simulink model "FMS_TECS"  (R2022b)
settings: Solver=FixedStepDiscrete  StartTime=0.0  StopTime=10.0  FixedStep=CONTROL_CONST.dt  RelTol=1e-3
values from neighbouring files (symbols this model uses):
  CONTROL_PARAM = Simulink.Parameter(CONTROL_PARAM_VALUE)    [control_model_init.m]
undefined symbols (not defined in the file or in its folder): CONTROL_CONST, CONTROL_PARAM_VALUE, DiscIntNeverNeededParam
libraries: FC_Lib x5, simulink x1, aerolibasang x1
settings Model: Creator=19114  LastModifiedBy=19114
settings OptimizationCC: DefaultParameterBehavior=Inlined  DefaultUnderspecifiedDataType=single  EnhancedBackFolding=on  PassReuseOutputArgsAs=Individual arguments  ZeroExternalMemoryAtStartup=off  ZeroInternalMemoryAtStartup=off  OptimizeBlockOrder=speed  DifferentSizesBufferReuse=on  OptimizationCustomize=off  EfficientTunableParamExpr=on
settings DebuggingCC: ParameterTunabilityLossMsg=error
settings HardwareCC: ProdBitPerLong=64  ProdLongLongMode=on  ProdHWDeviceType=Intel->x86-64 (Linux 64)
settings SFSimCC: MATLABDynamicMemAlloc=off
settings RTWCC: Description=Embedded Coder  SystemTargetFile=ert.tlc  GenCodeOnly=on  TemplateMakefile=ert_default_tmf  TargetLang=C++
settings CodeAppCC: ForceParamTrailComments=on  IgnoreCustomStorageClasses=off  OperatorAnnotations=on  SimulinkDataObjDesc=on  SFDataObjDesc=on  InsertBlockDesc=on
settings ERTTargetCC: TargetLangStandard=C++11 (ISO)  GenerateSampleERTMain=on  CodeInterfacePackaging=C++ class  InlinedParameterPlacement=NonHierarchical  RootIOFormat=Structure reference  ERTCustomFileTemplate=example_file_process.tlc

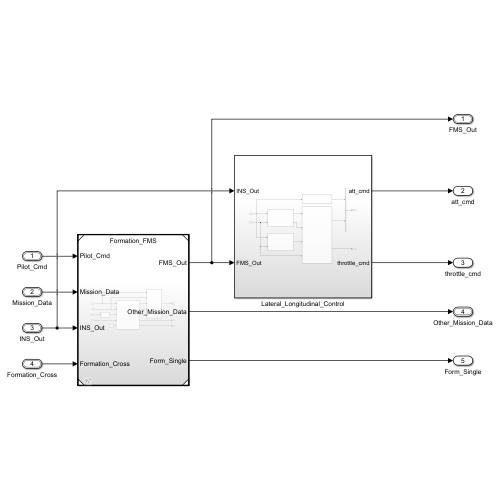
[thumbnail: Simulink's stored preview of the top-level diagram]
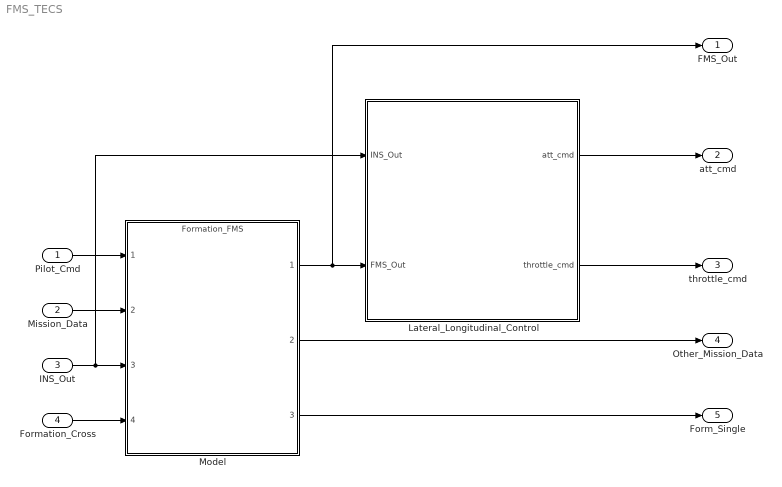
== system FMS_TECS ==
  Pilot_Cmd : Inport  OutDataTypeStr=Bus: Pilot_Cmd_Bus
  Mission_Data : Inport  Port=2  OutDataTypeStr=Bus: Mission_Data_Bus
  INS_Out : Inport  Port=3  OutDataTypeStr=Bus: INS_Out_Bus
  Formation_Cross : Inport  Port=4  OutDataTypeStr=Bus: Formation_Cross_Bus
  Lateral_Longitudinal_Control : Subsystem
  Model : ModelReference  ModelNameDialog=Formation_FMS.slx  SimulationMode=Normal  ModelReferenceVersion=1.179
  FMS_Out : Outport  OutDataTypeStr=Bus: FMS_Out_Bus  VectorParamsAs1DForOutWhenUnconnected=off
  att_cmd : Outport  Port=2
  throttle_cmd : Outport  Port=3
  Other_Mission_Data : Outport  Port=4  OutDataTypeStr=Bus: Other_Mission_Data_Bus  VectorParamsAs1DForOutWhenUnconnected=off
  Form_Single : Outport  Port=5
  wires:
  Lateral_Longitudinal_Control/1(att_cmd) -> att_cmd/1
  Lateral_Longitudinal_Control/2(throttle_cmd) -> throttle_cmd/1
  Pilot_Cmd/1 -> Model/1
  Mission_Data/1 -> Model/2
  INS_Out/1 -> Lateral_Longitudinal_Control/1(INS_Out), Model/3
  Formation_Cross/1 -> Model/4
  Model/1 -> FMS_Out/1, Lateral_Longitudinal_Control/2(FMS_Out)
  Model/2 -> Other_Mission_Data/1
  Model/3 -> Form_Single/1

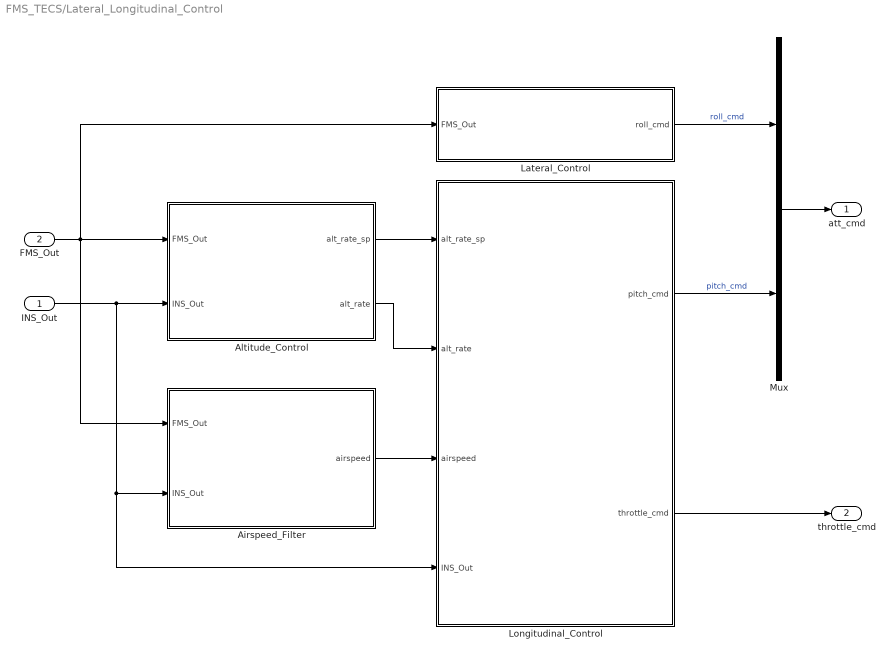
== system FMS_TECS/Lateral_Longitudinal_Control ==
  INS_Out : Inport
  FMS_Out : Inport  Port=2
  Airspeed_Filter : Subsystem
  Altitude_Control : Subsystem
  Lateral_Control : Subsystem
  Longitudinal_Control : Subsystem
  Mux : Mux  Inputs=2
  att_cmd : Outport  VectorParamsAs1DForOutWhenUnconnected=off
  throttle_cmd : Outport  Port=2  VectorParamsAs1DForOutWhenUnconnected=off
  wires:
  FMS_Out/1 -> Lateral_Control/1(FMS_Out), Airspeed_Filter/1(FMS_Out), Altitude_Control/1(FMS_Out)
  Altitude_Control/1(alt_rate_sp) -> Longitudinal_Control/1(alt_rate_sp)
  INS_Out/1 -> Longitudinal_Control/4(INS_Out), Airspeed_Filter/2(INS_Out), Altitude_Control/2(INS_Out)
  Longitudinal_Control/1(pitch_cmd) -> Mux/2  "pitch_cmd"
  Altitude_Control/2(alt_rate) -> Longitudinal_Control/2(alt_rate)
  Longitudinal_Control/2(throttle_cmd) -> throttle_cmd/1
  Airspeed_Filter/1(airspeed) -> Longitudinal_Control/3(airspeed)
  Lateral_Control/1(roll_cmd) -> Mux/1  "roll_cmd"
  Mux/1 -> att_cmd/1

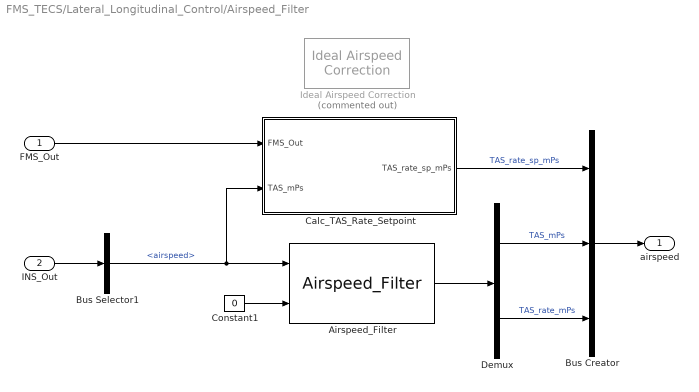
== system FMS_TECS/Lateral_Longitudinal_Control/Airspeed_Filter ==
  FMS_Out : Inport
  INS_Out : Inport  Port=2
  Airspeed_Filter : FC_Lib/Control/Airspeed_Filter
      settings: SourceProductName=Flight Control Toolbox
  Bus Creator : BusCreator  Inputs=3
  Bus Selector1 : BusSelector  OutputSignals=airspeed
  Calc_TAS_Rate_Setpoint : Subsystem
  Constant1 : Constant  Value=0  OutDataTypeStr=single
  Demux : Demux  Outputs=2
  Ideal Airspeed Correction : aerolibasang/Ideal Airspeed Correction  Commented=on  units=Metric (MKS)  vel_in=CAS  vel_out_tas=CAS  vel_out_eas=TAS  vel_out_cas=TAS  method=Table Lookup  SubOnly=on  action=None
  airspeed : Outport
  wires:
  INS_Out/1 -> Bus Selector1/1
  Bus Creator/1 -> airspeed/1
  Bus Selector1/1 -> Calc_TAS_Rate_Setpoint/2(TAS_mPs), Airspeed_Filter/1  "<airspeed>"
  FMS_Out/1 -> Calc_TAS_Rate_Setpoint/1(FMS_Out)
  Calc_TAS_Rate_Setpoint/1(TAS_rate_sp_mPs) -> Bus Creator/1  "TAS_rate_sp_mPs"
  Demux/1 -> Bus Creator/2  "TAS_mPs"
  Demux/2 -> Bus Creator/3  "TAS_rate_mPs"
  Airspeed_Filter/1 -> Demux/1
  Constant1/1 -> Airspeed_Filter/2

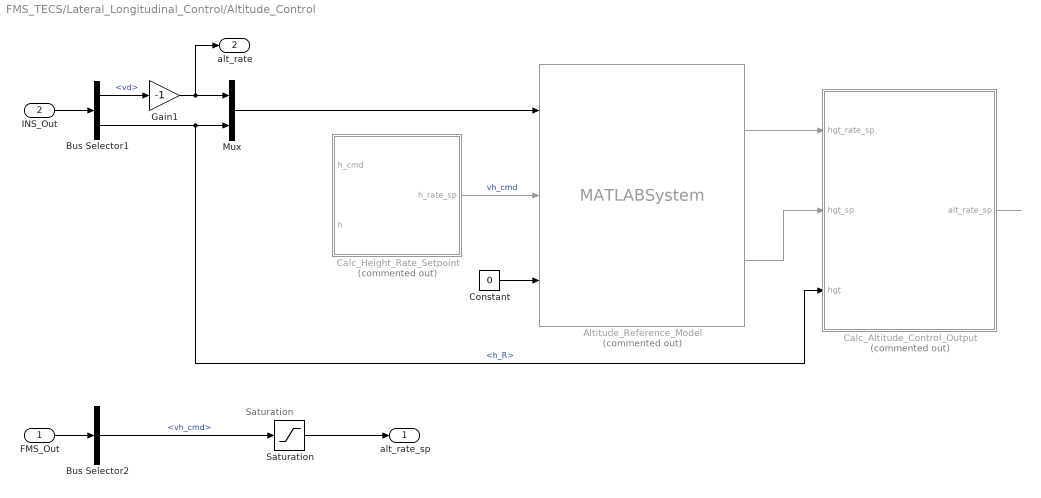
== system FMS_TECS/Lateral_Longitudinal_Control/Altitude_Control ==
  note: Saturation
  FMS_Out : Inport
  INS_Out : Inport  Port=2
  Altitude_Reference_Model : MATLABSystem  Commented=on  System=VelocitySmoothing  max_jerk=single(1000)  max_accel=CONTROL_PARAM.FW_T_VERT_ACC  max_climb_rate=CONTROL_PARAM.FW_T_CLMB_MAX  max_sink_rate=CONTROL_PARAM.FW_T_SINK_MAX  SampleTime=CONTROL_CONST.dt  SimulateUsing=Code generation
      mask Type: VelocitySmoothing
      mask Display:
      | disp(['Velocity' char(10) 'Smoothing']);
      | port_label('input',1,'v0x0');
      | port_label('input',2,'vel_sp');
      | port_label('input',3,'reset');
      | port_label('output',1,'vel');
      | port_label('output',2,'pos');
  Bus Selector1 : BusSelector  OutputSignals=vd,h_R
  Bus Selector2 : BusSelector  OutputSignals=vh_cmd
  Calc_Altitude_Control_Output : Subsystem  Commented=on
  Calc_Height_Rate_Setpoint : Subsystem  Commented=on
  Constant : Constant  Value=0  OutDataTypeStr=single
  Gain1 : Gain  Gain=-1
  Mux : Mux  Inputs=2
  Saturation : Saturate  UpperLimit=CONTROL_PARAM.FW_T_CLMB_MAX  LowerLimit=-CONTROL_PARAM.FW_T_SINK_MAX
  alt_rate_sp : Outport
  alt_rate : Outport  Port=2
  wires:
  FMS_Out/1 -> Bus Selector2/1
  INS_Out/1 -> Bus Selector1/1
  Bus Selector1/2 -> Mux/2, Calc_Altitude_Control_Output/3(hgt)  "<h_R>"
  Bus Selector2/1 -> Saturation/1  "<vh_cmd>"
  Bus Selector1/1 -> Gain1/1  "<vd>"
  Gain1/1 -> Mux/1, alt_rate/1
  Mux/1 -> Altitude_Reference_Model/1
  Altitude_Reference_Model/2 -> Calc_Altitude_Control_Output/2(hgt_sp)
  Constant/1 -> Altitude_Reference_Model/3
  Altitude_Reference_Model/1 -> Calc_Altitude_Control_Output/1(hgt_rate_sp)
  Calc_Altitude_Control_Output/1(alt_rate_sp) -> ?
  Calc_Height_Rate_Setpoint/1(h_rate_sp) -> Altitude_Reference_Model/2  "vh_cmd"
  Saturation/1 -> alt_rate_sp/1

== system FMS_TECS/Lateral_Longitudinal_Control/Lateral_Control ==
  FMS_Out : Inport
  Atan : Trigonometry  Operator=atan
  Bus Selector : BusSelector  OutputSignals=ay_cmd
  Constant : Constant  Value=CONTROL_CONST.g
  Product : Product  Inputs=/*
  Saturation : Saturate  UpperLimit=CONTROL_PARAM.FW_R_LIM  LowerLimit=-CONTROL_PARAM.FW_R_LIM
  roll_cmd : Outport
  wires:
  FMS_Out/1 -> Bus Selector/1
  Constant/1 -> Product/1
  Bus Selector/1 -> Product/2  "<ay_cmd>"
  Product/1 -> Atan/1
  Atan/1 -> Saturation/1
  Saturation/1 -> roll_cmd/1

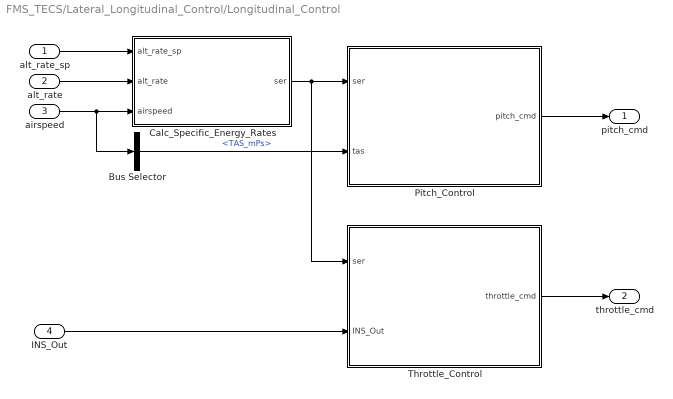
== system FMS_TECS/Lateral_Longitudinal_Control/Longitudinal_Control ==
  alt_rate_sp : Inport
  alt_rate : Inport  Port=2
  airspeed : Inport  Port=3
  INS_Out : Inport  Port=4
  Bus Selector : BusSelector  OutputSignals=TAS_mPs
  Calc_Specific_Energy_Rates : Subsystem
  Pitch_Control : Subsystem
  Throttle_Control : Subsystem
  pitch_cmd : Outport
  throttle_cmd : Outport  Port=2
  wires:
  alt_rate_sp/1 -> Calc_Specific_Energy_Rates/1(alt_rate_sp)
  alt_rate/1 -> Calc_Specific_Energy_Rates/2(alt_rate)
  Throttle_Control/1(throttle_cmd) -> throttle_cmd/1
  Pitch_Control/1(pitch_cmd) -> pitch_cmd/1
  INS_Out/1 -> Throttle_Control/2(INS_Out)
  Calc_Specific_Energy_Rates/1(ser) -> Pitch_Control/1(ser), Throttle_Control/1(ser)
  Bus Selector/1 -> Pitch_Control/2(tas)  "<TAS_mPs>"
  airspeed/1 -> Bus Selector/1, Calc_Specific_Energy_Rates/3(airspeed)

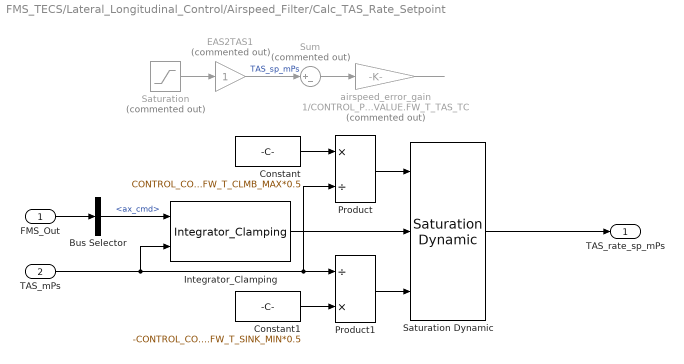
== system FMS_TECS/Lateral_Longitudinal_Control/Airspeed_Filter/Calc_TAS_Rate_Setpoint ==
  FMS_Out : Inport
  TAS_mPs : Inport  Port=2
  Bus Selector : BusSelector  OutputSignals=ax_cmd
  Constant : Constant  Value=CONTROL_CONST.g*CONTROL_PARAM.FW_T_CLMB_MAX*0.5  OutDataTypeStr=single
  Constant1 : Constant  Value=-CONTROL_CONST.g*CONTROL_PARAM.FW_T_SINK_MIN*0.5  OutDataTypeStr=single
  EAS2TAS1 : Gain  Commented=on
  Integrator_Clamping : FC_Lib/Control/Integrator_Clamping  uplimit=CONTROL_PARAM.FW_AIRSPD_MAX  downlimit=CONTROL_PARAM.FW_AIRSPD_MIN
      settings: LibrarySourceBlock=|
      | simulink/User-Defined
      | Functions/MATLAB Function
  Product : Product  Inputs=*/
  Product1 : Product  Inputs=/*
  Saturation : Saturate  Commented=on  UpperLimit=CONTROL_PARAM.FW_AIRSPD_MAX  LowerLimit=CONTROL_PARAM.FW_AIRSPD_MIN
  Saturation Dynamic : simulink/Discontinuities/Saturation Dynamic  OutMin=[]  OutMax=[]  OutDataTypeStr=Inherit: Same as second input  OutDataType=fixdt(1, 16)  OutScaling=2^-10  DoSatur=off
  Sum : Sum  Commented=on  Inputs=|+-
  airspeed_error_gain : Gain  Commented=on  Gain=1/CONTROL_PARAM_VALUE.FW_T_TAS_TC
  TAS_rate_sp_mPs : Outport
  wires:
  Saturation Dynamic/1 -> TAS_rate_sp_mPs/1
  Sum/1 -> airspeed_error_gain/1
  FMS_Out/1 -> Bus Selector/1
  airspeed_error_gain/1 -> ?
  Constant/1 -> Product/1
  Product/1 -> Saturation Dynamic/1
  Product1/1 -> Saturation Dynamic/3
  Constant1/1 -> Product1/2
  ? -> Saturation/1  "u_cmd"
  EAS2TAS1/1 -> Sum/1  "TAS_sp_mPs"
  Saturation/1 -> EAS2TAS1/1
  Bus Selector/1 -> Integrator_Clamping/1  "<ax_cmd>"
  Integrator_Clamping/1 -> Saturation Dynamic/2
  TAS_mPs/1 -> Integrator_Clamping/2, Product/2, Product1/1

== system FMS_TECS/Lateral_Longitudinal_Control/Altitude_Control/Calc_Altitude_Control_Output ==
  note: Saturation
  hgt_rate_sp : Inport
  hgt_sp : Inport  Port=2
  hgt : Inport  Port=3
  Gain : Gain  Gain=CONTROL_PARAM.FW_T_HRATE_FF
  Gain2 : Gain  Gain=1/max(CONTROL_PARAM.FW_T_ALT_TC,0.1)
  Saturation : Saturate  UpperLimit=CONTROL_PARAM.FW_T_CLMB_MAX  LowerLimit=-CONTROL_PARAM.FW_T_SINK_MAX
  Sum : Sum  Inputs=|++
  Sum1 : Sum  Inputs=|+-
  alt_rate_sp : Outport
  wires:
  Sum1/1 -> Gain2/1
  hgt_sp/1 -> Sum1/1
  Gain/1 -> Sum/1  "alt_rate_gain_ff"
  hgt_rate_sp/1 -> Gain/1
  hgt/1 -> Sum1/2
  Sum/1 -> Saturation/1
  Gain2/1 -> Sum/2  "alt_gain"
  Saturation/1 -> alt_rate_sp/1

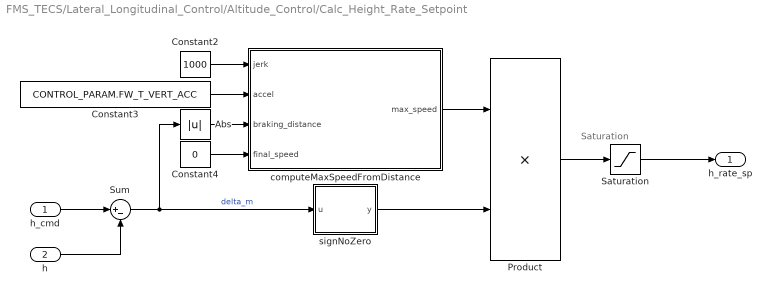
== system FMS_TECS/Lateral_Longitudinal_Control/Altitude_Control/Calc_Height_Rate_Setpoint ==
  note: Saturation
  h_cmd : Inport
  h : Inport  Port=2
  Abs : Abs  SaturateOnIntegerOverflow=off
  Constant2 : Constant  Value=1000  OutDataTypeStr=single
  Constant3 : Constant  Value=CONTROL_PARAM.FW_T_VERT_ACC  OutDataTypeStr=single
  Constant4 : Constant  Value=0  OutDataTypeStr=single
  Product : Product
  Saturation : Saturate  UpperLimit=min(CONTROL_PARAM.FW_T_CLMB_R_SP, CONTROL_PARAM.FW_T_CLMB_MAX)  LowerLimit=-min(CONTROL_PARAM.FW_T_SINK_R_SP, CONTROL_PARAM.FW_T_SINK_MAX)
  Sum : Sum  Inputs=|+-  OutDataTypeStr=Inherit: Same as first input
  computeMaxSpeedFromDistance : MATLAB Function  TreatAsAtomicUnit=on
  signNoZero : MATLAB Function  TreatAsAtomicUnit=on
  h_rate_sp : Outport  OutDataTypeStr=single
  wires:
  computeMaxSpeedFromDistance/1(max_speed) -> Product/1
  Constant3/1 -> computeMaxSpeedFromDistance/2(accel)
  h/1 -> Sum/2
  Sum/1 -> Abs/1, signNoZero/1(u)  "delta_m"
  Abs/1 -> computeMaxSpeedFromDistance/3(braking_distance)
  Constant2/1 -> computeMaxSpeedFromDistance/1(jerk)
  Constant4/1 -> computeMaxSpeedFromDistance/4(final_speed)
  signNoZero/1(y) -> Product/2
  h_cmd/1 -> Sum/1
  Product/1 -> Saturation/1
  Saturation/1 -> h_rate_sp/1

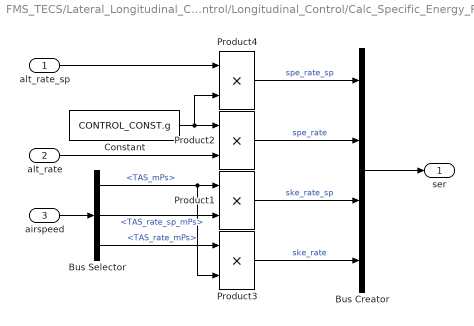
== system FMS_TECS/Lateral_Longitudinal_Control/Longitudinal_Control/Calc_Specific_Energy_Rates ==
  alt_rate_sp : Inport
  alt_rate : Inport  Port=2
  airspeed : Inport  Port=3
  Bus Creator : BusCreator  Inputs=4
  Bus Selector : BusSelector  OutputSignals=TAS_mPs,TAS_rate_sp_mPs,TAS_rate_mPs
  Constant : Constant  Value=CONTROL_CONST.g
  Product{1..4} (4 alike) : Product
  ser : Outport
  wires:
  Product4/1 -> Bus Creator/1  "spe_rate_sp"
  airspeed/1 -> Bus Selector/1
  Bus Selector/1 -> Product3/2, Product1/1  "<TAS_mPs>"
  Bus Selector/2 -> Product1/2  "<TAS_rate_sp_mPs>"
  Product1/1 -> Bus Creator/3  "ske_rate_sp"
  Bus Selector/3 -> Product3/1  "<TAS_rate_mPs>"
  Product2/1 -> Bus Creator/2  "spe_rate"
  Product3/1 -> Bus Creator/4  "ske_rate"
  Bus Creator/1 -> ser/1
  Constant/1 -> Product4/2, Product2/1
  alt_rate/1 -> Product2/2
  alt_rate_sp/1 -> Product4/1

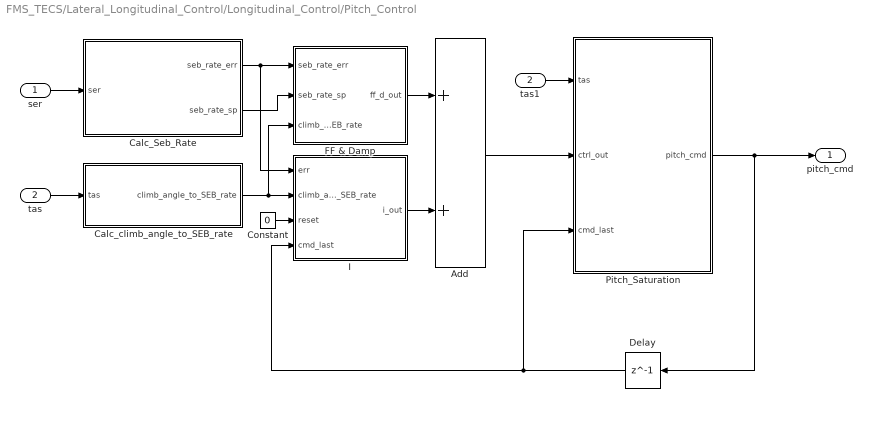
== system FMS_TECS/Lateral_Longitudinal_Control/Longitudinal_Control/Pitch_Control ==
  ser : Inport
  tas : Inport  Port=2
  Add : Sum
  Calc_Seb_Rate : Subsystem
  Calc_climb_angle_to_SEB_rate : Subsystem
  Constant : Constant  Value=0  OutDataTypeStr=single
  Delay : Delay  DelayLength=1
  FF & Damp : Subsystem
  I : Subsystem
  Pitch_Saturation : Subsystem
  tas1 : InportShadow  Port=2
  pitch_cmd : Outport
  wires:
  ser/1 -> Calc_Seb_Rate/1(ser)
  Calc_Seb_Rate/1(seb_rate_err) -> I/1(err), FF & Damp/1(seb_rate_err)
  I/1(i_out) -> Add/2
  Delay/1 -> I/4(cmd_last), Pitch_Saturation/3(cmd_last)
  Calc_Seb_Rate/2(seb_rate_sp) -> FF & Damp/2(seb_rate_sp)
  FF & Damp/1(ff_d_out) -> Add/1
  Pitch_Saturation/1(pitch_cmd) -> pitch_cmd/1, Delay/1
  Add/1 -> Pitch_Saturation/2(ctrl_out)
  Constant/1 -> I/3(reset)
  tas/1 -> Calc_climb_angle_to_SEB_rate/1(tas)
  Calc_climb_angle_to_SEB_rate/1(climb_angle_to_SEB_rate) -> FF & Damp/3(climb_angle_to_SEB_rate), I/2(climb_angle_to_SEB_rate)
  tas1/1 -> Pitch_Saturation/1(tas)

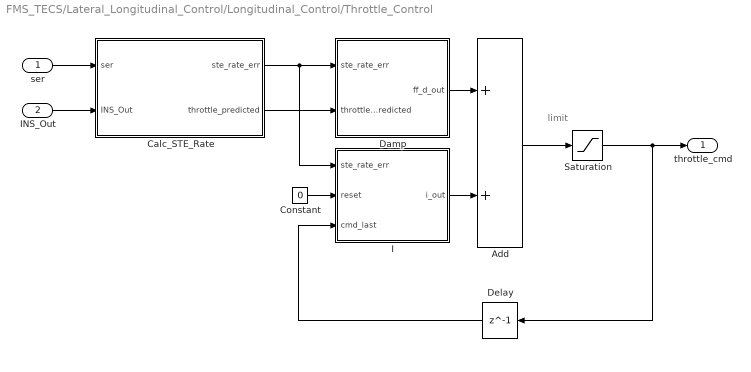
== system FMS_TECS/Lateral_Longitudinal_Control/Longitudinal_Control/Throttle_Control ==
  note: limit
  ser : Inport
  INS_Out : Inport  Port=2
  Add : Sum
  Calc_STE_Rate : Subsystem
  Constant : Constant  Value=0  OutDataTypeStr=single
  Damp : Subsystem
  Delay : Delay  DelayLength=1
  I : Subsystem
  Saturation : Saturate  UpperLimit=CONTROL_PARAM.FW_THR_MAX  LowerLimit=CONTROL_PARAM.FW_THR_MIN
  throttle_cmd : Outport
  wires:
  ser/1 -> Calc_STE_Rate/1(ser)
  I/1(i_out) -> Add/2
  Delay/1 -> I/3(cmd_last)
  Add/1 -> Saturation/1
  Calc_STE_Rate/2(throttle_predicted) -> Damp/2(throttle_predicted)
  Saturation/1 -> throttle_cmd/1, Delay/1
  Calc_STE_Rate/1(ste_rate_err) -> Damp/1(ste_rate_err), I/1(ste_rate_err)
  Damp/1(ff_d_out) -> Add/1
  Constant/1 -> I/2(reset)
  INS_Out/1 -> Calc_STE_Rate/2(INS_Out)

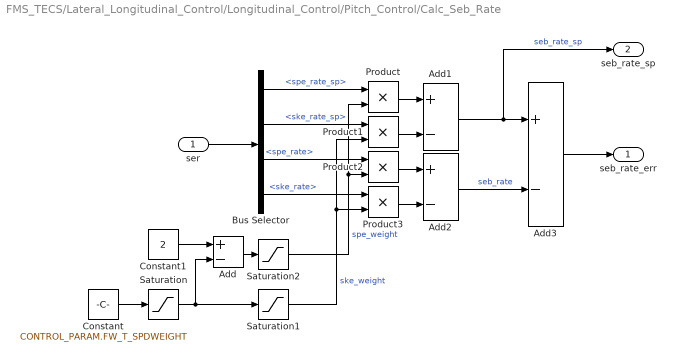
== system FMS_TECS/Lateral_Longitudinal_Control/Longitudinal_Control/Pitch_Control/Calc_Seb_Rate ==
  ser : Inport
  Add{,1..3} (4 alike) : Sum  Inputs=+-
  Bus Selector : BusSelector  OutputSignals=spe_rate_sp,ske_rate_sp,spe_rate,ske_rate
  Constant : Constant  Value=CONTROL_PARAM.FW_T_SPDWEIGHT  OutDataTypeStr=single
  Constant1 : Constant  Value=2  OutDataTypeStr=single
  Product{,1..3} (4 alike) : Product
  Saturation : Saturate  UpperLimit=2  LowerLimit=0
  Saturation1 : Saturate  UpperLimit=1  LowerLimit=0
  Saturation2 : Saturate  UpperLimit=1  LowerLimit=0
  seb_rate_err : Outport
  seb_rate_sp : Outport  Port=2
  wires:
  Saturation2/1 -> Product2/2, Product/2  "spe_weight"
  Add/1 -> Saturation2/1
  Saturation/1 -> Add/2, Saturation1/1
  Saturation1/1 -> Product1/2, Product3/2  "ske_weight"
  Constant1/1 -> Add/1
  Constant/1 -> Saturation/1
  ser/1 -> Bus Selector/1
  Bus Selector/1 -> Product/1  "<spe_rate_sp>"
  Bus Selector/2 -> Product1/1  "<ske_rate_sp>"
  Bus Selector/3 -> Product2/1  "<spe_rate>"
  Bus Selector/4 -> Product3/1  "<ske_rate>"
  Product1/1 -> Add1/2
  Product/1 -> Add1/1
  Product2/1 -> Add2/1
  Product3/1 -> Add2/2
  Add1/1 -> seb_rate_sp/1, Add3/1  "seb_rate_sp"
  Add2/1 -> Add3/2  "seb_rate"
  Add3/1 -> seb_rate_err/1

== system FMS_TECS/Lateral_Longitudinal_Control/Longitudinal_Control/Pitch_Control/Calc_climb_angle_to_SEB_rate ==
  tas : Inport
  Constant1 : Constant  Value=CONTROL_CONST.g
  Product : Product
  climb_angle_to_SEB_rate : Outport
  wires:
  Constant1/1 -> Product/1
  Product/1 -> climb_angle_to_SEB_rate/1
  tas/1 -> Product/2

== system FMS_TECS/Lateral_Longitudinal_Control/Longitudinal_Control/Pitch_Control/FF & Damp ==
  seb_rate_err : Inport
  seb_rate_sp : Inport  Port=2
  climb_angle_to_SEB_rate : Inport  Port=3
  Add : Sum
  Divide : Product  Inputs=*/
  pitch_damping_gain : Gain  Gain=CONTROL_PARAM.FW_T_PTCH_DAMP
  seb_rate_ff : Gain  Gain=CONTROL_PARAM.FW_T_SEB_R_FF
  ff_d_out : Outport
  wires:
  seb_rate_err/1 -> pitch_damping_gain/1
  seb_rate_sp/1 -> seb_rate_ff/1
  pitch_damping_gain/1 -> Add/1
  seb_rate_ff/1 -> Add/2
  Add/1 -> Divide/1
  climb_angle_to_SEB_rate/1 -> Divide/2
  Divide/1 -> ff_d_out/1

== system FMS_TECS/Lateral_Longitudinal_Control/Longitudinal_Control/Pitch_Control/I ==
  err : Inport
  climb_angle_to_SEB_rate : Inport  Port=2
  reset : Inport  Port=3
  cmd_last : Inport  Port=4
  Discrete-Time Integrator : DiscreteIntegrator  gainval=1  ExternalReset=level  SampleTime=-1  ICPrevOutput=DiscIntNeverNeededParam  ICPrevScaledInput=DiscIntNeverNeededParam
  Divide : Product  Inputs=*/
  I_Gain : Gain  Gain=CONTROL_PARAM.FW_T_I_GAIN_PIT
  Integrator_Clamping : FC_Lib/Control/Integrator_Clamping  uplimit=CONTROL_PARAM.FW_P_LIM_MAX  downlimit=CONTROL_PARAM.FW_P_LIM_MIN
      settings: LibrarySourceBlock=|
      | simulink/User-Defined
      | Functions/MATLAB Function
  i_out : Outport
  wires:
  Discrete-Time Integrator/1 -> i_out/1
  err/1 -> Divide/1
  cmd_last/1 -> Integrator_Clamping/2
  Integrator_Clamping/1 -> I_Gain/1
  reset/1 -> Discrete-Time Integrator/2
  climb_angle_to_SEB_rate/1 -> Divide/2
  Divide/1 -> Integrator_Clamping/1
  I_Gain/1 -> Discrete-Time Integrator/1

== system FMS_TECS/Lateral_Longitudinal_Control/Longitudinal_Control/Pitch_Control/Pitch_Saturation ==
  note: saturation
  tas : Inport
  ctrl_out : Inport  Port=2
  cmd_last : Inport  Port=3
  Pitch_Saturation : MATLAB Function  TreatAsAtomicUnit=on  mask{limit=CONTROL_PARAM.FW_T_VERT_ACC}
      mask prompts: limit "vert_accel_limit"
  Saturation : Saturate  UpperLimit=CONTROL_PARAM.FW_P_LIM_MAX  LowerLimit=CONTROL_PARAM.FW_P_LIM_MIN
  Weighted Sample Time : SampleTimeMath  TsampMathOp=Ts Only
  pitch_cmd : Outport
  wires:
  ctrl_out/1 -> Saturation/1
  cmd_last/1 -> Pitch_Saturation/3(y_last)
  Saturation/1 -> Pitch_Saturation/1(u)
  tas/1 -> Pitch_Saturation/2(tas)
  Weighted Sample Time/1 -> Pitch_Saturation/4(dt)
  Pitch_Saturation/1(y) -> pitch_cmd/1

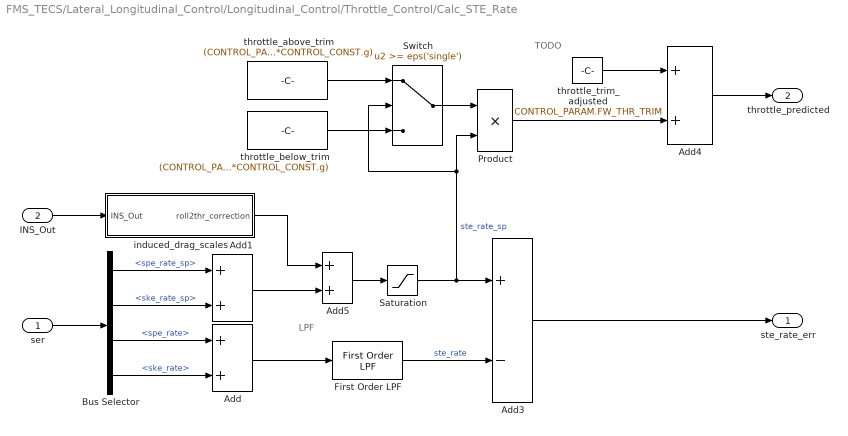
== system FMS_TECS/Lateral_Longitudinal_Control/Longitudinal_Control/Throttle_Control/Calc_STE_Rate ==
  note: TODO
  note: LPF
  ser : Inport
  INS_Out : Inport  Port=2
  Add{,1,4..5} (4 alike) : Sum
  Add3 : Sum  Inputs=+-
  Bus Selector : BusSelector  OutputSignals=spe_rate_sp,ske_rate_sp,spe_rate,ske_rate
  First Order LPF : FC_Lib/Filter/First Order LPF  fc=1/(2*pi*0.4)
      settings: SourceProductName=Flight Control Toolbox
  Product : Product
  Saturation : Saturate  UpperLimit=CONTROL_PARAM.FW_T_CLMB_MAX*CONTROL_CONST.g  LowerLimit=-CONTROL_PARAM.FW_T_SINK_MIN*CONTROL_CONST.g
  Switch : Switch  Threshold=eps('single')  SaturateOnIntegerOverflow=off  InputSameDT=off
  induced_drag_scales : Subsystem
  throttle_above_trim : Constant  Value=(CONTROL_PARAM.FW_THR_MAX-CONTROL_PARAM.FW_THR_TRIM)/(CONTROL_PARAM.FW_T_CLMB_MAX*CONTROL_CONST.g)
  throttle_below_trim : Constant  Value=(CONTROL_PARAM.FW_THR_TRIM-CONTROL_PARAM.FW_THR_MIN)/(CONTROL_PARAM.FW_T_SINK_MIN*CONTROL_CONST.g)
  throttle_trim_adjusted : Constant  Value=CONTROL_PARAM.FW_THR_TRIM  OutDataTypeStr=single
  ste_rate_err : Outport
  throttle_predicted : Outport  Port=2
  wires:
  Bus Selector/3 -> Add/1  "<spe_rate>"
  Bus Selector/2 -> Add1/2  "<ske_rate_sp>"
  Add1/1 -> Add5/2
  Bus Selector/4 -> Add/2  "<ske_rate>"
  Bus Selector/1 -> Add1/1  "<spe_rate_sp>"
  ser/1 -> Bus Selector/1
  Add/1 -> First Order LPF/1
  Saturation/1 -> Switch/2, Product/2, Add3/1  "ste_rate_sp"
  Add3/1 -> ste_rate_err/1
  throttle_below_trim/1 -> Switch/3
  throttle_above_trim/1 -> Switch/1
  Switch/1 -> Product/1
  throttle_trim_adjusted/1 -> Add4/1
  Product/1 -> Add4/2
  Add4/1 -> throttle_predicted/1
  Add5/1 -> Saturation/1
  INS_Out/1 -> induced_drag_scales/1(INS_Out)
  induced_drag_scales/1(roll2thr_correction) -> Add5/1
  First Order LPF/1 -> Add3/2  "ste_rate"

== system FMS_TECS/Lateral_Longitudinal_Control/Longitudinal_Control/Throttle_Control/Damp ==
  ste_rate_err : Inport
  throttle_predicted : Inport  Port=2
  Add : Sum
  Product : Product
  STE_rate_to_throttle : Constant  Value=1/(CONTROL_CONST.g*(CONTROL_PARAM.FW_T_CLMB_MAX+CONTROL_PARAM.FW_T_SINK_MAX))
  throttle_damping_gain : Gain  Gain=CONTROL_PARAM.FW_T_THR_DAMP
  ff_d_out : Outport
  wires:
  ste_rate_err/1 -> throttle_damping_gain/1
  throttle_damping_gain/1 -> Product/1
  throttle_predicted/1 -> Add/2
  Add/1 -> ff_d_out/1
  Product/1 -> Add/1
  STE_rate_to_throttle/1 -> Product/2

== system FMS_TECS/Lateral_Longitudinal_Control/Longitudinal_Control/Throttle_Control/I ==
  ste_rate_err : Inport
  reset : Inport  Port=2
  cmd_last : Inport  Port=3
  Discrete-Time Integrator : DiscreteIntegrator  gainval=1  ExternalReset=level  SampleTime=-1  ICPrevOutput=DiscIntNeverNeededParam  ICPrevScaledInput=DiscIntNeverNeededParam
  I_Gain : Gain  Gain=CONTROL_PARAM.FW_T_I_GAIN_THR
  Integrator_Clamping : FC_Lib/Control/Integrator_Clamping  uplimit=CONTROL_PARAM.FW_THR_MAX  downlimit=CONTROL_PARAM.FW_THR_MIN
      settings: LibrarySourceBlock=|
      | simulink/User-Defined
      | Functions/MATLAB Function
  Product : Product
  STE_rate_to_throttle : Constant  Value=1/(CONTROL_CONST.g*(CONTROL_PARAM.FW_T_CLMB_MAX+CONTROL_PARAM.FW_T_SINK_MAX))
  i_out : Outport
  wires:
  Discrete-Time Integrator/1 -> i_out/1
  cmd_last/1 -> Integrator_Clamping/2
  ste_rate_err/1 -> Product/1
  STE_rate_to_throttle/1 -> Product/2
  Integrator_Clamping/1 -> I_Gain/1
  Product/1 -> Integrator_Clamping/1
  reset/1 -> Discrete-Time Integrator/2
  I_Gain/1 -> Discrete-Time Integrator/1

== system FMS_TECS/Lateral_Longitudinal_Control/Longitudinal_Control/Throttle_Control/Calc_STE_Rate/induced_drag_scales ==
  INS_Out : Inport
  Bias : Bias  Bias=-1  SaturateOnIntegerOverflow=off
  Bus Selector1 : BusSelector  OutputSignals=phi
  Constant1 : Constant  OutDataTypeStr=single
  Cos : Trigonometry  Operator=cos
  Divide3 : Product  Inputs=*/
  load_factor_correction : Gain  Gain=CONTROL_PARAM.FW_T_RLL2THR
  roll2thr_correction : Outport
  wires:
  INS_Out/1 -> Bus Selector1/1
  Bus Selector1/1 -> Cos/1  "<phi>"
  Constant1/1 -> Divide3/1
  Cos/1 -> Divide3/2
  Divide3/1 -> Bias/1
  Bias/1 -> load_factor_correction/1
  load_factor_correction/1 -> roll2thr_correction/1

== matlab function FMS_TECS/Lateral_Longitudinal_Control/Longitudinal_Control/Pitch_Control/Pitch_Saturation/Pitch_Saturation ==
  data: u input; tas input; y output; limit parameter; y_last input; dt input
function y = fcn(u, tas, limit, y_last, dt)
pitch_increment = dt * limit / max(tas, eps('like', tas));
u_min = y_last - pitch_increment;
u_max = y_last + pitch_increment;

if u < u_min
    y = u_min;
else 
    if u > u_max
        y = u_max;
    else
        y = u;
    end
end

== matlab function FMS_TECS/Lateral_Longitudinal_Control/Altitude_Control/Calc_Height_Rate_Setpoint/signNoZero ==
  data: u input; y output
function y = fcn(u)

y = cast((0 <= u) - (u < 0), 'like', u);

== matlab function FMS_TECS/Lateral_Longitudinal_Control/Altitude_Control/Calc_Height_Rate_Setpoint/computeMaxSpeedFromDistance ==
  data: jerk input; max_speed output; accel input; braking_distance input; final_speed input
function max_speed = fcn(jerk, accel, braking_distance, final_speed)
    sqr = @(f) f * f;
    b = 4.0 * sqr(accel) / jerk;
    c = -2.0 * accel * braking_distance - sqr(final_speed);
    max_speed = 0.5 * (-b + sqrt(sqr(b) - 4.0 * c));
    
    % 不要减速超过最终速度，即使保守的加速度请求时间要求减速更多
    max_speed = max(max_speed, final_speed);
end
